simulink model "simulinkBlockLibraryTest"  (Simulink 8.9)
settings: Solver=ode3  StartTime=0.0  StopTime=3  FixedStep=jObj.Ts_elec  RelTol=1e-3
values from neighbouring files (symbols this model uses):
  jObj = elTestJointStatic    [cjtJointBuilderTest.m]    (also in cjtSimulinkLibraryTest.m = testCase.('TestData').testJoint; simulinkLibraryTest.m = testCase.('TestData').testJoint)
undefined symbols (not defined in the file or in its folder): DiscIntNeverNeededParam
libraries: cjt_library_models x2
settings Model: SuppressorTable=22 serialization::archive 11 0 6 0 0 0 11 0  Creator=joern  LastModifiedBy=wesley
settings DataIOCC: LimitDataPoints=off  SignalLoggingSaveFormat=Dataset
settings DebuggingCC: UnderspecifiedInitializationDetection=Simplified  MergeDetectMultiDrivingBlocksExec=error  SolverPrmCheckMsg=warning  FcnCallInpInsideContextMsg=error  StateNameClashWarn=none
settings GRTTargetCC: CombineOutputUpdateFcns=on  GRTInterface=off
settings ConfigComp: CovSFcnEnable=off

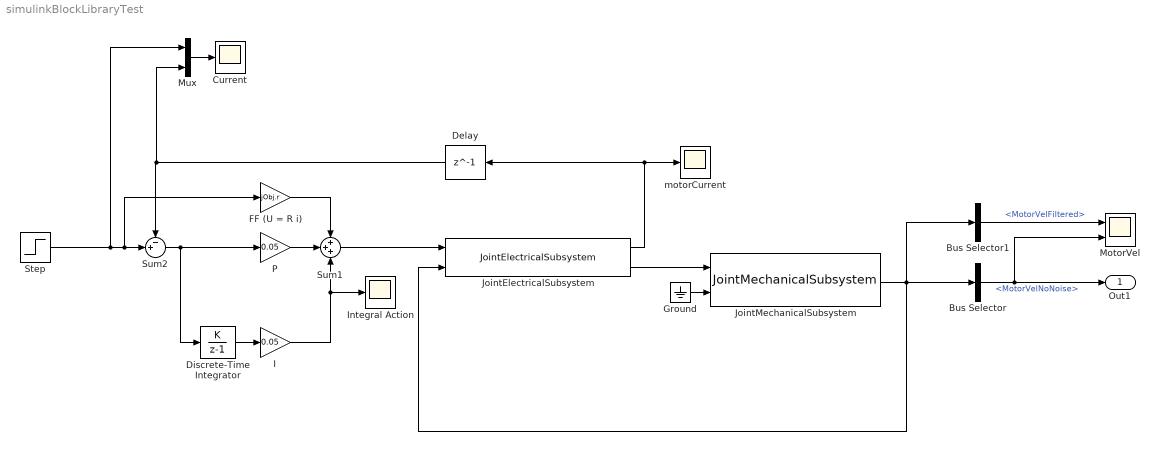
== system simulinkBlockLibraryTest ==
  Bus Selector : BusSelector  OutputSignals=MotorVelNoNoise
  Bus Selector1 : BusSelector  OutputSignals=MotorVelFiltered
  Current : Scope
  Delay : Delay  DelayLength=1  InitialCondition=0  SampleTime=jObj.Ts_elec
  Discrete-Time Integrator : DiscreteIntegrator  IntegratorMethod=Accumulation: Forward Euler  SampleTime=jObj.Ts  ICPrevOutput=DiscIntNeverNeededParam  ICPrevScaledInput=DiscIntNeverNeededParam
  FF (U = R i) : Gain  Gain=jObj.r
  Ground : Ground
  I : Gain  Gain=0.05
  Integral Action : Scope
  JointElectricalSubsystem : cjt_library_models/Joint models/JointElectricalSubsystem  jointObj=jObj  input_delay=0  quantize=off  quantize_bits=32  input_noise_enabled=off  var_u=0.12
  JointMechanicalSubsystem : cjt_library_models/Joint models/JointMechanicalSubsystem  jointObj=jObj  fc_vel=499  fc_torque=499  input_delay=0  output_delay=0  quantize=off  quantize_bits=19  input_noise_enabled=off  output_noise_enabled=off  var_u=0.12^2  var_y=1.8e-10
  MotorVel : Scope  NumInputPorts=2
  Mux : Mux  Inputs=2
  P : Gain  Gain=0.05
  Step : Step  SampleTime=jObj.Ts
  Sum1 : Sum  Inputs=+++
  Sum2 : Sum  Inputs=-+|
  motorCurrent : Scope
  Out1 : Outport
  wires:
  I/1 -> Sum1/3, Integral Action/1
  Sum2/1 -> Discrete-Time Integrator/1, P/1
  Discrete-Time Integrator/1 -> I/1
  Mux/1 -> Current/1
  JointElectricalSubsystem/1 -> motorCurrent/1, Delay/1
  Step/1 -> Mux/1, FF (U = R i)/1, Sum2/2
  Sum1/1 -> JointElectricalSubsystem/1
  Bus Selector/1 -> MotorVel/2, Out1/1  "<MotorVelNoNoise>"
  Ground/1 -> JointMechanicalSubsystem/2
  JointMechanicalSubsystem/1 -> Bus Selector1/1, JointElectricalSubsystem/2, Bus Selector/1
  Delay/1 -> Mux/2, Sum2/1
  P/1 -> Sum1/2
  FF (U = R i)/1 -> Sum1/1
  JointElectricalSubsystem/2 -> JointMechanicalSubsystem/1
  Bus Selector1/1 -> MotorVel/1  "<MotorVelFiltered>"
